simulink model "RTD"  (R2022b)
settings: Solver=VariableStepAuto  StartTime=0.0  StopTime=120  RelTol=1e-3
undefined symbols (not defined in the file): v
libraries: Solver_SF x1
settings Model: Creator=ASOAT  LastModifiedBy=ASOAT

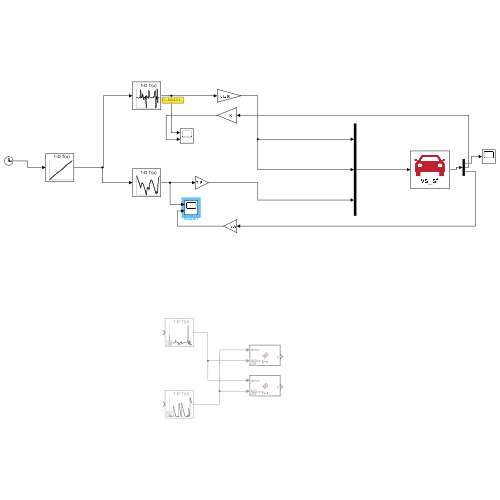
[thumbnail: Simulink's stored preview of the top-level diagram]
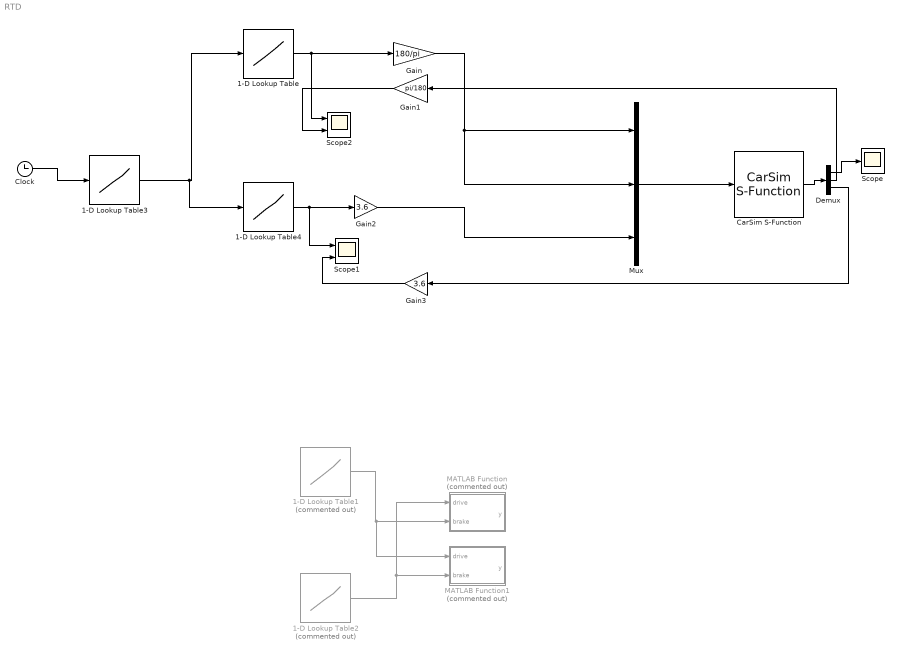
== system RTD ==
  1-D Lookup Table : Lookup_n-D  NumberOfTableDimensions=1  BreakpointsForDimension1=u(:,1)  Table=u(:,2)  InternalRulePriority=Speed  RndMeth=Simplest
  1-D Lookup Table1 : Lookup_n-D  Commented=on  NumberOfTableDimensions=1  BreakpointsForDimension1=u(:,1)  Table=u(:,3)  InternalRulePriority=Speed  RndMeth=Simplest
  1-D Lookup Table2 : Lookup_n-D  Commented=on  NumberOfTableDimensions=1  BreakpointsForDimension1=u(:,1)  Table=u(:,4)  InternalRulePriority=Speed  RndMeth=Simplest
  1-D Lookup Table3 : Lookup_n-D  NumberOfTableDimensions=1  BreakpointsForDimension1=t(:,2)  Table=t(:,1)  InternalRulePriority=Speed  RndMeth=Simplest
  1-D Lookup Table4 : Lookup_n-D  NumberOfTableDimensions=1  BreakpointsForDimension1=v(:,1)  Table=v(:,2)  InternalRulePriority=Speed  RndMeth=Simplest
  CarSim S-Function : Solver_SF/CarSim S-Function  Priority=1  SIMFILE=simfile.sim  Run_RTs=off  vs_state_ind=Run  StopMode_ind=Vehicle Model
  Clock : Clock
  Demux : Demux  Outputs=3
  Gain : Gain  Gain=180/pi
  Gain1 : Gain  Gain=pi/180
  Gain2 : Gain  Gain=3.6
  Gain3 : Gain  Gain=3.6
  MATLAB Function : MATLAB Function  Commented=on  TreatAsAtomicUnit=on
  MATLAB Function1 : MATLAB Function  Commented=on  TreatAsAtomicUnit=on
  Mux : Mux  Inputs=3
  Scope : Scope
  Scope1 : Scope  NumInputPorts=2
  Scope2 : Scope  NumInputPorts=2
  wires:
  Mux/1 -> CarSim S-Function/1
  1-D Lookup Table2/1 -> MATLAB Function/1(drive), MATLAB Function1/2(brake)
  1-D Lookup Table1/1 -> MATLAB Function1/1(drive), MATLAB Function/2(brake)
  Gain/1 -> Mux/2, Mux/1
  1-D Lookup Table/1 -> Gain/1, Scope2/1
  Clock/1 -> 1-D Lookup Table3/1
  1-D Lookup Table3/1 -> 1-D Lookup Table4/1, 1-D Lookup Table/1
  CarSim S-Function/1 -> Demux/1
  Demux/1 -> Scope/1
  Demux/2 -> Gain1/1
  Gain1/1 -> Scope2/2
  1-D Lookup Table4/1 -> Scope1/1, Gain2/1
  Gain2/1 -> Mux/3
  Demux/3 -> Gain3/1
  Gain3/1 -> Scope1/2

== matlab function RTD/MATLAB Function ==
  data: drive input; brake input; y output
function y = fcn(drive, brake)

if brake > 1.0
    y = 0.6 * brake;
else
    y = 0 * drive;
end

== matlab function RTD/MATLAB Function1 ==
  data: drive input; brake input; y output
function y = fcn(drive, brake)

if brake > 1.0
    y = 0.4 * brake;
else
    y =  drive;
end
